simulink subsystem "subsysSensores"  (R2023b)
settings: Solver=VariableStepAuto  StartTime=0.0  StopTime=10.0  RelTol=1e-3
libraries: arduinolib x2
settings Model: Creator=Pedro  LastModifiedBy=Pedro

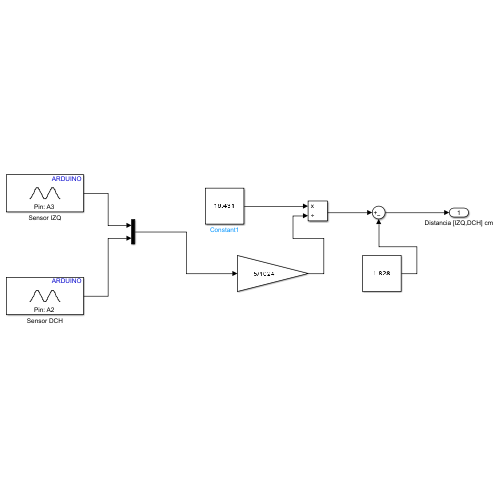
[thumbnail: Simulink's stored preview of the top-level diagram]
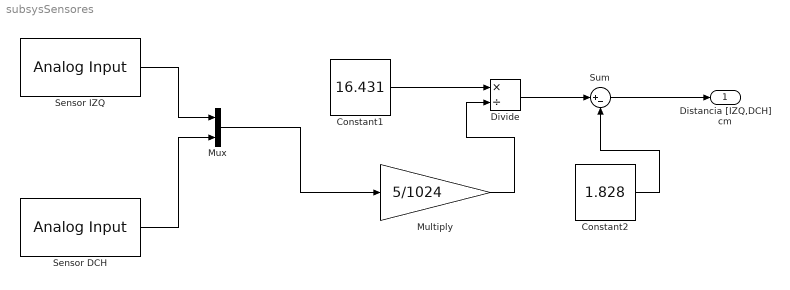
== system subsysSensores ==
  Constant1 : Constant  Value=16.431
  Constant2 : Constant  Value=1.828
  Divide : Product  Inputs=*/
  Multiply : Gain  Gain=5/1024
  Mux : Mux  Inputs=2
  Sensor DCH : arduinolib/Analog Input  pinNumber=2  ReadResultsOnly=off  ConversionTriggerSource=Software  ExternalTriggerType=uint32( 0 )  OutputDataType=uint16  EnableConversionCompleteNotify=off  EnableOuputStatus=off  SampleTime=-1  blockPlatform=arduino
  Sensor IZQ : arduinolib/Analog Input  pinNumber=3  ReadResultsOnly=off  ConversionTriggerSource=Software  ExternalTriggerType=uint32( 0 )  OutputDataType=uint16  EnableConversionCompleteNotify=off  EnableOuputStatus=off  SampleTime=-1  blockPlatform=arduino
  Sum : Sum  Inputs=|+-
  Distancia [IZQ,DCH] cm : Outport
  wires:
  Sensor DCH/1 -> Mux/2
  Mux/1 -> Multiply/1
  Divide/1 -> Sum/1
  Sum/1 -> Distancia [IZQ,DCH] cm/1
  Multiply/1 -> Divide/2
  Constant2/1 -> Sum/2
  Sensor IZQ/1 -> Mux/1
  Constant1/1 -> Divide/1
